simulink model "sampleModel1699"  (R2023a)
settings: Solver=VariableStepAuto  StartTime=0.0  StopTime=10.0  RelTol=1e-3
libraries: hdlsllib x6, simulink x2
settings Model: Creator=user1  LastModifiedBy=user1

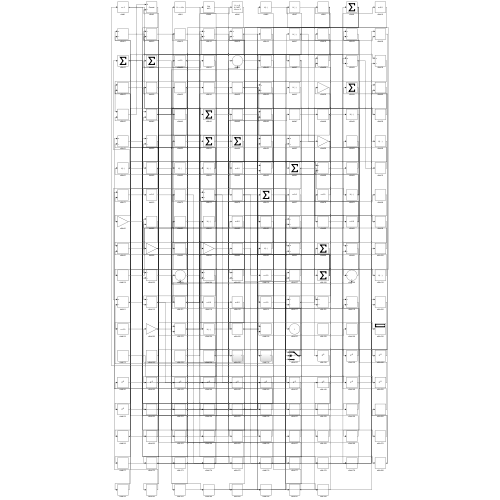
[thumbnail: Simulink's stored preview of the top-level diagram]
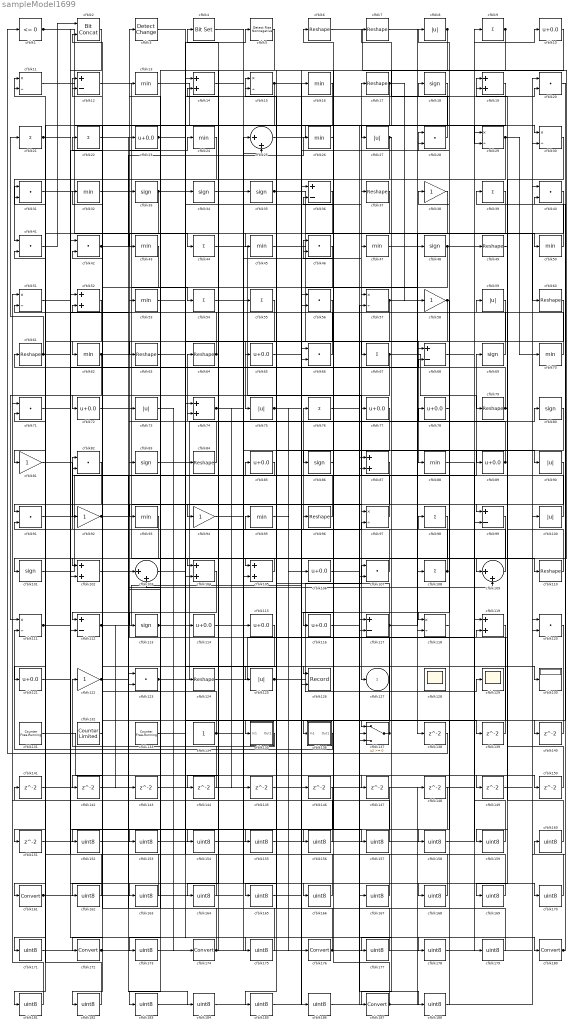
== system sampleModel1699 ==
  cfblk1 : hdlsllib/Logic and Bit Operations/Compare To Zero  relop=<=  OutDataTypeStr=boolean
  cfblk{10,23,65,72,77..78,85,89,106,114..116,121} (13 alike) : Bias  Bias=0.0  SaturateOnIntegerOverflow=off
  cfblk{8,27,59,73,75,90,100,125} (8 alike) : Abs  SaturateOnIntegerOverflow=off
  cfblk{18,33..35,48,69,80,83,86,101,113} (11 alike) : Signum
  cfblk{14,19,52,74,87,102,104..105,119} (9 alike) : Sum
  cfblk103 : Sum  Inputs=|++
  cfblk{20,28,31,40..42,46,56,66,71,82,91,107,120,123} (15 alike) : DotProduct  OutDataTypeStr=Inherit: Inherit via internal rule
  cfblk{9,21..22,39,44,54..55,67,76,98,108} (11 alike) : Sum  Inputs=+
  cfblk109 : Sum  Inputs=|++
  cfblk{11,15,29..30,51,57,97,111,118} (9 alike) : Product  Inputs=*/  RndMeth=Zero  SaturateOnIntegerOverflow=on
  cfblk{6..7,17,37,49,60..61,63..64,79,84,96,110,124} (14 alike) : Reshape
  cfblk{12,36,68,99,112,117} (6 alike) : Sum  Inputs=+-
  cfblk{38,58,81,92,94,122} (6 alike) : Gain
  cfblk126 : Record  FileSettingsInternal="{\"entries\":[{\"content\":{\"excelSettings\":{\"content\":{},\"type\":\"Streamout.ExcelSettings\"}},\"type\":\"Streamout.FileSettingStorage\",\"uuid\":\"\"}],\"packageUris\":[\"http:\\/\\/schema.mathworks.com\\/mf0\\/streamout_blocks\\/R2020a\"],\"version\":\"1.0\"}"  Layout=[1 1]  SignalsInternal="{\"entries\":[{\"content\":{\"signals\":[{\"content\":{\"blockPath\":[],\"dimensions\":[1],\"domain\":\"\",\"lineColor\":\"#a2142f\",\"plots\":[1],\"port\":1,\"signalID\":3065,\"signalName\":\"XY Graph:1\"},\"type\":\"RecordBlkView.Signal\",\"uuid\":\"\"},{\"content\":{\"blockPath\":[],\"dimensions\":[1],\"domain\":\"\",\"lineColor\":\"#139fff\",\"plots\":[1],\"port\":2,\"signalID\":3068,\"signalName\":\"XY Graph:2\"},\"type\":\"RecordBlkView.Signal\",\"uuid\":\"\"}]},\"type\":\"RecordBlkView.InputSignals\",\"uuid\":\"\"}],\"packageUris\":[\"http:\\/\\/schema.mathworks.com\\/mf0\\/streamout_blocks\\/R2020a\"],\"version\":\"1.0\"}"  VisualizationBindings="{\"xyplotplugin\":{\"info\":[{\"series\":[{\"bindingParametersList\":[{\"parameter\":\"X-Axis\",\"signalID\":3065,\"signalName\":\"XY Graph:1\"},{\"parameter\":\"Y-Axis\",\"signalID\":3068,\"signalName\":\"XY Graph:2\"}],\"seriesID\":25029}],\"subplotID\":1}]}}"  CompatibilityTag=XY  st=-1
  cfblk128 : Scope
      settings: Floating=on
  cfblk129 : Scope
  cfblk{13,16,24,26,32,43,45,47,50,53,62,70,88,93,95} (15 alike) : MinMax
  cfblk130 : Display
  cfblk131 : hdlsllib/Sources/Counter Free-Running  NumBits=16  tsamp=-1
  cfblk132 : hdlsllib/Sources/Counter Limited  uplimit=7  tsamp=-1
  cfblk133 : hdlsllib/Sources/Counter Free-Running  NumBits=16  tsamp=-1
  cfblk134 : Constant  SampleTime=-1
  cfblk135 : Subsystem
      settings: LibrarySourceBlock=|
      | hdlsllib/Ports &
      | Subsystems/Subsystem
  cfblk136 : Subsystem
      settings: LibrarySourceBlock=|
      | hdlsllib/Ports &
      | Subsystems/Subsystem
  cfblk137 : Switch  SaturateOnIntegerOverflow=off  InputSameDT=off
  cfblk{138..151} (14 alike) : Delay  SampleTime=1
  cfblk{152..160,162..171,173,175,177..179,181..186,188} (31 alike) : DataTypeConversion  OutDataTypeStr=uint8  SaturateOnIntegerOverflow=off  RndMeth=Floor
  cfblk{161,172,174,176,180,187} (6 alike) : DataTypeConversion  SaturateOnIntegerOverflow=off  RndMeth=Floor
  cfblk2 : hdlsllib/Logic and Bit Operations/Bit Concat  numInputs=2
  cfblk25 : Sum  Inputs=|++
  cfblk3 : simulink/Logic and Bit Operations/Detect Change  vinit=0  OutDataTypeStr=boolean
      settings: LibrarySourceBlock=|
      | hdlsllib/Logic and Bit
      | Operations/Detect
      | Change
  cfblk4 : simulink/Logic and Bit Operations/Bit Set  iBit=0
      settings: LibrarySourceBlock=|
      | hdlsllib/Logic and Bit
      | Operations/Bit Set
  cfblk5 : hdlsllib/Logic and Bit Operations/Detect Rise Nonnegative  vinit=0  OutDataTypeStr=boolean
  cfblk127 : Outport  VectorParamsAs1DForOutWhenUnconnected=off
  wires:
  cfblk17/1 -> cfblk58/1, cfblk66/2
  cfblk29/1 -> cfblk70/1, cfblk125/1
  cfblk80/1 -> cfblk101/1
  cfblk62/1 -> cfblk111/1, cfblk168/1
  cfblk108/1 -> cfblk82/1, cfblk91/2, cfblk36/2
  cfblk60/1 -> cfblk75/1
  cfblk6/1 -> cfblk109/1
  cfblk44/1 -> cfblk127/1
  cfblk91/1 -> cfblk3/1
  cfblk41/1 -> cfblk2/1
  cfblk89/1 -> cfblk64/1, cfblk8/1
  cfblk46/1 -> cfblk112/1
  cfblk95/1 -> cfblk176/1
  cfblk100/1 -> cfblk17/1
  cfblk28/1 -> cfblk7/1
  cfblk10/1 -> cfblk45/1
  cfblk61/1 -> cfblk21/1, cfblk68/2
  cfblk112/1 -> cfblk36/1, cfblk143/1
  cfblk101/1 -> cfblk69/1
  cfblk111/1 -> cfblk24/1, cfblk11/2
  cfblk8/1 -> cfblk27/1, cfblk126/2
  cfblk12/1 -> cfblk110/1
  cfblk99/1 -> cfblk117/2
  cfblk118/1 -> cfblk38/1
  cfblk48/1 -> cfblk49/1, cfblk103/2
  cfblk51/1 -> cfblk180/1
  cfblk117/1 -> cfblk48/1, cfblk15/2, cfblk182/1
  cfblk35/1 -> cfblk88/1, cfblk60/1
  cfblk18/1 -> cfblk72/1
  cfblk133/1 -> cfblk34/1
  cfblk123/1 -> cfblk77/1, cfblk37/1
  cfblk57/1 -> cfblk90/1, cfblk165/1
  cfblk98/1 -> cfblk187/1
  cfblk135/1(Out1) -> cfblk122/1
  cfblk110/1 -> cfblk19/1
  cfblk77/1 -> cfblk105/1
  cfblk9/1 -> cfblk65/1, cfblk113/1, cfblk86/1
  cfblk105/1 -> cfblk104/1
  cfblk81/1 -> cfblk92/1
  cfblk73/1 -> cfblk174/1
  cfblk68/1 -> cfblk10/1
  cfblk58/1 -> cfblk94/1, cfblk118/1
  cfblk85/1 -> cfblk82/2
  cfblk137/1 -> cfblk33/1, cfblk96/1
  cfblk125/1 -> cfblk107/1, cfblk129/1
  cfblk11/1 -> cfblk114/1
  cfblk113/1 -> cfblk84/1, cfblk97/2, cfblk20/2
  cfblk90/1 -> cfblk102/1
  cfblk70/1 -> cfblk6/1
  cfblk65/1 -> cfblk28/1
  cfblk42/1 -> cfblk54/1, cfblk44/1, cfblk26/1
  cfblk26/1 -> cfblk116/1
  cfblk121/1 -> cfblk53/1
  cfblk37/1 -> cfblk136/1(In1)
  cfblk19/1 -> cfblk43/1
  cfblk25/1 -> cfblk30/1
  cfblk30/1 -> cfblk99/1
  cfblk39/1 -> cfblk104/2
  cfblk4/1 -> cfblk105/2
  cfblk50/1 -> cfblk39/1
  cfblk1/1 -> cfblk29/2, cfblk157/1
  cfblk75/1 -> cfblk106/1, cfblk147/1
  cfblk96/1 -> cfblk15/1
  cfblk13/1 -> cfblk137/3
  cfblk16/1 -> cfblk112/2
  cfblk23/1 -> cfblk93/1, cfblk126/1
  cfblk92/1 -> cfblk2/2, cfblk149/1
  cfblk122/1 -> cfblk85/1, cfblk12/2
  cfblk109/1 -> cfblk13/1
  cfblk124/1 -> cfblk9/1
  cfblk72/1 -> cfblk97/1
  cfblk107/1 -> cfblk76/1
  cfblk114/1 -> cfblk130/1
  cfblk27/1 -> cfblk41/1, cfblk67/1
  cfblk136/1(Out1) -> cfblk111/2
  cfblk69/1 -> cfblk18/1
  cfblk15/1 -> cfblk118/2, cfblk151/1
  cfblk115/1 -> cfblk172/1
  cfblk82/1 -> cfblk121/1
  cfblk78/1 -> cfblk28/2
  cfblk66/1 -> cfblk31/1
  cfblk94/1 -> cfblk80/1
  cfblk24/1 -> cfblk63/1
  cfblk3/1 -> cfblk124/1
  cfblk47/1 -> cfblk50/1
  cfblk103/1 -> cfblk135/1(In1)
  cfblk134/1 -> cfblk22/1, cfblk46/1
  cfblk2/1 -> cfblk102/2
  cfblk132/1 -> cfblk12/1
  cfblk67/1 -> cfblk79/1, cfblk81/1
  cfblk84/1 -> cfblk23/1
  cfblk74/1 -> cfblk47/1, cfblk145/1
  cfblk34/1 -> cfblk55/1
  cfblk21/1 -> cfblk163/1, cfblk175/1
  cfblk79/1 -> cfblk59/1, cfblk57/1, cfblk61/1
  cfblk45/1 -> cfblk108/1
  cfblk64/1 -> cfblk41/2, cfblk11/1
  cfblk97/1 -> cfblk4/1
  cfblk33/1 -> cfblk5/1, cfblk123/2
  cfblk22/1 -> cfblk109/2
  cfblk31/1 -> cfblk74/1
  cfblk38/1 -> cfblk91/1
  cfblk63/1 -> cfblk68/1
  cfblk54/1 -> cfblk89/1
  cfblk43/1 -> cfblk62/1
  cfblk52/1 -> cfblk161/1
  cfblk7/1 -> cfblk138/1
  cfblk138/1 -> cfblk1/1
  cfblk53/1 -> cfblk139/1
  cfblk139/1 -> cfblk117/1
  cfblk20/1 -> cfblk140/1
  cfblk140/1 -> cfblk137/1
  cfblk141/1 -> cfblk29/1
  cfblk104/1 -> cfblk142/1
  cfblk142/1 -> cfblk137/2
  cfblk143/1 -> cfblk25/2
  cfblk36/1 -> cfblk144/1
  cfblk144/1 -> cfblk103/1
  cfblk149/1 -> cfblk30/2
  cfblk116/1 -> cfblk150/1
  cfblk150/1 -> cfblk19/2
  cfblk151/1 -> cfblk99/2
  cfblk56/1 -> cfblk152/1
  cfblk152/1 -> cfblk25/1
  cfblk148/1 -> cfblk153/1
  cfblk153/1 -> cfblk56/1
  cfblk5/1 -> cfblk154/1
  cfblk154/1 -> cfblk56/2
  cfblk71/1 -> cfblk155/1
  cfblk155/1 -> cfblk16/1
  cfblk86/1 -> cfblk156/1
  cfblk156/1 -> cfblk71/1
  cfblk157/1 -> cfblk71/2
  cfblk119/1 -> cfblk158/1
  cfblk158/1 -> cfblk78/1
  cfblk49/1 -> cfblk159/1
  cfblk159/1 -> cfblk119/1
  cfblk160/1 -> cfblk119/2
  cfblk161/1 -> cfblk35/1, cfblk31/2
  cfblk147/1 -> cfblk162/1
  cfblk162/1 -> cfblk52/1
  cfblk163/1 -> cfblk52/2
  cfblk146/1 -> cfblk164/1
  cfblk164/1 -> cfblk42/2
  cfblk165/1 -> cfblk146/1
  cfblk14/1 -> cfblk166/1
  cfblk166/1 -> cfblk42/1
  cfblk76/1 -> cfblk167/1
  cfblk167/1 -> cfblk14/1
  cfblk168/1 -> cfblk14/2
  cfblk120/1 -> cfblk169/1
  cfblk169/1 -> cfblk141/1
  cfblk32/1 -> cfblk170/1
  cfblk170/1 -> cfblk120/1
  cfblk59/1 -> cfblk171/1
  cfblk171/1 -> cfblk120/2
  cfblk172/1 -> cfblk57/2, cfblk107/2
  cfblk55/1 -> cfblk173/1
  cfblk173/1 -> cfblk115/1
  cfblk174/1 -> cfblk74/2, cfblk123/1
  cfblk175/1 -> cfblk73/1
  cfblk176/1 -> cfblk32/1, cfblk20/1
  cfblk40/1 -> cfblk177/1
  cfblk177/1 -> cfblk95/1
  cfblk83/1 -> cfblk178/1
  cfblk178/1 -> cfblk40/1
  cfblk88/1 -> cfblk179/1
  cfblk179/1 -> cfblk83/1
  cfblk180/1 -> cfblk160/1, cfblk40/2
  cfblk93/1 -> cfblk181/1
  cfblk181/1 -> cfblk51/1
  cfblk182/1 -> cfblk51/2
  cfblk87/1 -> cfblk183/1
  cfblk183/1 -> cfblk66/1
  cfblk102/1 -> cfblk184/1
  cfblk184/1 -> cfblk87/1
  cfblk145/1 -> cfblk185/1
  cfblk185/1 -> cfblk87/2
  cfblk131/1 -> cfblk186/1
  cfblk186/1 -> cfblk100/1
  cfblk187/1 -> cfblk148/1, cfblk46/2
  cfblk106/1 -> cfblk188/1
  cfblk188/1 -> cfblk98/1

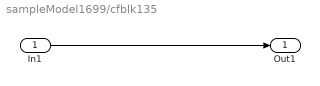
== system sampleModel1699/cfblk135 ==
  In1 : Inport
  Out1 : Outport
  wires:
  In1/1 -> Out1/1

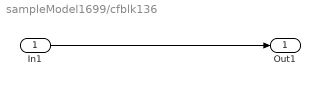
== system sampleModel1699/cfblk136 ==
  In1 : Inport
  Out1 : Outport
  wires:
  In1/1 -> Out1/1
